simulink model "arm_model_pid"  (Simulink 7.7)
settings: Solver=ode4  StartTime=0.0  StopTime=1  FixedStep=1e-3  RelTol=1e-3
values from neighbouring files (symbols this model uses):
  dest = find_ik_solution(target,[L1,L2])    [init_param.m]
  g = 9.81    [init_param.m]    (also in nms_model_MechInit.m)
  L1 = 0.28    [init_param.m]
  L2 = 0.32    [init_param.m]
  N = 1.5    [muscleParams.m]    (also in nms_model_MechInit.m)
  s = orProblemSendCommand(['LoadIKFastSolver robot Translation3D'],probid)    [init.m]
libraries: mblibv1 x17, simulink x5
settings Model: Creator=icoderaven  LastModifiedBy=icoderaven
settings DataIOCC: SignalLoggingSaveFormat=Dataset
settings OptimizationCC: ExpressionDepthLimit=128
settings DebuggingCC: FcnCallInpInsideContextMsg=Enable All
settings CodeAppCC: CustomSymbolStrType=$N$R$M_T
settings GRTTargetCC: CombineOutputUpdateFcns=on
settings SimMechanicsCC: VisOnUpdateDiagram=on  VisDuringSimulation=on
settings ConfigurationSet: Description=SimMechanics 2G

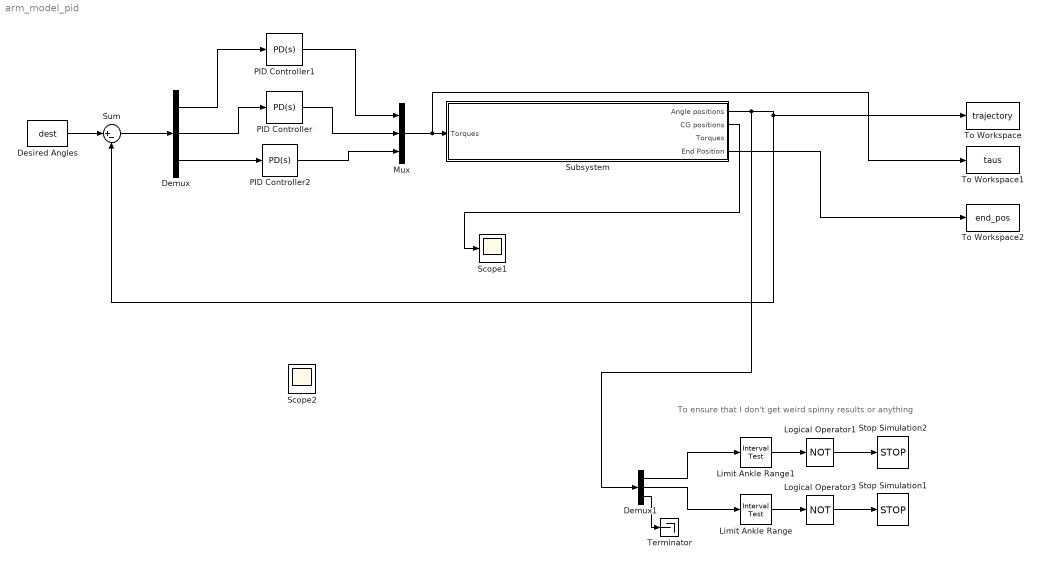
== system arm_model_pid ==
  note: To ensure that I don't get weird spinny results or anything
  Demux : Demux  Outputs=3
  Demux1 : Demux  Outputs=3
  Desired Angles : Constant  Value=dest
  Limit Ankle Range : simulink/Logic and Bit Operations/Interval Test  IntervalClosedRight=on  uplimit=150*pi/180  IntervalClosedLeft=on  lowlimit=0*pi/180  LogicOutDataTypeMode=boolean
  Limit Ankle Range1 : simulink/Logic and Bit Operations/Interval Test  IntervalClosedRight=on  uplimit=180*pi/180  IntervalClosedLeft=on  lowlimit=-45*pi/180  LogicOutDataTypeMode=boolean
  Logical Operator1 : Logic  Operator=NOT  AllPortsSameDT=off  OutDataTypeStr=boolean
  Logical Operator3 : Logic  Operator=NOT  AllPortsSameDT=off  OutDataTypeStr=boolean
  Mux : Mux  Inputs=3
  PID Controller : simulink/Continuous/PID Controller  Controller=PD  TimeDomain=Continuous-time  SampleTime=1  IntegratorMethod=Forward Euler  FilterMethod=Forward Euler  Form=Parallel  P=34.6616213286309  I=0.219466074591108  D=6.99160554908179  N=51.5441934181628  InitialConditionSource=internal  InitialConditionForIntegrator=0  InitialConditionForFilter=0  ExternalReset=none  LimitOutput=on  UpperSaturationLimit=200  LowerSaturationLimit=-200  LinearizeAsGain=off  AntiWindupMode=none  Kb=1  TrackingMode=off  Kt=1  PParamMin=[]  PParamMax=[]  IParamMin=[]  IParamMax=[]  DParamMin=[]  DParamMax=[]  NParamMin=[]  NParamMax=[]  KbParamMin=[]  KbParamMax=[]  KtParamMin=[]  KtParamMax=[]  POutMin=[]  POutMax=[]  IOutMin=[]  IOutMax=[]  DOutMin=[]  DOutMax=[]  NOutMin=[]  NOutMax=[]  KbOutMin=[]  KbOutMax=[]  KtOutMin=[]  KtOutMax=[]  IntegratorOutMin=[]  IntegratorOutMax=[]  FilterOutMin=[]  FilterOutMax=[]  SumOutMin=[]  SumOutMax=[]  SumI1OutMin=[]  SumI1OutMax=[]  SumI2OutMin=[]  SumI2OutMax=[]  SumI3OutMin=[]  SumI3OutMax=[]  SumDOutMin=[]  SumDOutMax=[]  SaturationOutMin=[]  SaturationOutMax=[]  IntegratorContinuousStateAttributes=''  IntegratorStateMustResolveToSignalObject=off  IntegratorRTWStateStorageClass=Auto  FilterContinuousStateAttributes=''  FilterStateMustResolveToSignalObject=off  FilterRTWStateStorageClass=Auto
  PID Controller1 : simulink/Continuous/PID Controller  Controller=PD  TimeDomain=Continuous-time  SampleTime=1  IntegratorMethod=Forward Euler  FilterMethod=Forward Euler  Form=Parallel  P=74.4712745992682  I=15180.7317223686  D=10.4723028081317  N=27.129113033617  InitialConditionSource=internal  InitialConditionForIntegrator=0  InitialConditionForFilter=0  ExternalReset=none  LimitOutput=on  UpperSaturationLimit=200  LowerSaturationLimit=-200  LinearizeAsGain=off  AntiWindupMode=none  Kb=1  TrackingMode=off  Kt=1  PParamMin=[]  PParamMax=[]  IParamMin=[]  IParamMax=[]  DParamMin=[]  DParamMax=[]  NParamMin=[]  NParamMax=[]  KbParamMin=[]  KbParamMax=[]  KtParamMin=[]  KtParamMax=[]  POutMin=[]  POutMax=[]  IOutMin=[]  IOutMax=[]  DOutMin=[]  DOutMax=[]  NOutMin=[]  NOutMax=[]  KbOutMin=[]  KbOutMax=[]  KtOutMin=[]  KtOutMax=[]  IntegratorOutMin=[]  IntegratorOutMax=[]  FilterOutMin=[]  FilterOutMax=[]  SumOutMin=[]  SumOutMax=[]  SumI1OutMin=[]  SumI1OutMax=[]  SumI2OutMin=[]  SumI2OutMax=[]  SumI3OutMin=[]  SumI3OutMax=[]  SumDOutMin=[]  SumDOutMax=[]  SaturationOutMin=[]  SaturationOutMax=[]  IntegratorContinuousStateAttributes=''  IntegratorStateMustResolveToSignalObject=off  IntegratorRTWStateStorageClass=Auto  FilterContinuousStateAttributes=''  FilterStateMustResolveToSignalObject=off  FilterRTWStateStorageClass=Auto
  PID Controller2 : simulink/Continuous/PID Controller  Controller=PD  TimeDomain=Continuous-time  SampleTime=1  IntegratorMethod=Forward Euler  FilterMethod=Forward Euler  Form=Parallel  P=5.74233404990851  I=38.1400991342515  D=65.6199753295884  N=1142.8279760416  InitialConditionSource=internal  InitialConditionForIntegrator=0  InitialConditionForFilter=0  ExternalReset=none  LimitOutput=on  UpperSaturationLimit=200  LowerSaturationLimit=-200  LinearizeAsGain=on  AntiWindupMode=none  Kb=1  TrackingMode=off  Kt=1  PParamMin=[]  PParamMax=[]  IParamMin=[]  IParamMax=[]  DParamMin=[]  DParamMax=[]  NParamMin=[]  NParamMax=[]  KbParamMin=[]  KbParamMax=[]  KtParamMin=[]  KtParamMax=[]  POutMin=[]  POutMax=[]  IOutMin=[]  IOutMax=[]  DOutMin=[]  DOutMax=[]  NOutMin=[]  NOutMax=[]  KbOutMin=[]  KbOutMax=[]  KtOutMin=[]  KtOutMax=[]  IntegratorOutMin=[]  IntegratorOutMax=[]  FilterOutMin=[]  FilterOutMax=[]  SumOutMin=[]  SumOutMax=[]  SumI1OutMin=[]  SumI1OutMax=[]  SumI2OutMin=[]  SumI2OutMax=[]  SumI3OutMin=[]  SumI3OutMax=[]  SumDOutMin=[]  SumDOutMax=[]  SaturationOutMin=[]  SaturationOutMax=[]  IntegratorContinuousStateAttributes=''  IntegratorStateMustResolveToSignalObject=off  IntegratorRTWStateStorageClass=Auto  FilterContinuousStateAttributes=''  FilterStateMustResolveToSignalObject=off  FilterRTWStateStorageClass=Auto
  Scope1 : Scope
      settings: YMin=-1.3  YMax=0  SaveName=ScopeData4
  Scope2 : Scope  NumInputPorts=6
      settings: YMin=-1.3~-5~-5~-5~-5~-5  YMax=0~5~5~5~5~5  SaveName=ScopeData5
  Stop Simulation1 : Stop
  Stop Simulation2 : Stop
  Subsystem : Subsystem
  Sum : Sum  Inputs=|+-
  Terminator : Terminator
  To Workspace : ToWorkspace  VariableName=trajectory  SampleTime=-1  SaveFormat=Structure With Time
  To Workspace1 : ToWorkspace  VariableName=taus  SampleTime=-1  SaveFormat=Structure With Time
  To Workspace2 : ToWorkspace  VariableName=end_pos  SampleTime=-1  SaveFormat=Structure With Time
  wires:
  Mux/1 -> To Workspace1/1, Subsystem/1("Torques ")
  Sum/1 -> Demux/1
  PID Controller/1 -> Mux/2
  Demux/3 -> PID Controller2/1
  Demux/2 -> PID Controller/1
  Demux/1 -> PID Controller1/1
  PID Controller1/1 -> Mux/1
  PID Controller2/1 -> Mux/3
  Subsystem/2("CG positions ") -> Scope1/1
  Desired Angles/1 -> Sum/1
  Subsystem/4(End Position) -> To Workspace2/1
  Subsystem/1(Angle positions) -> Demux1/1, Sum/2, To Workspace/1
  Limit Ankle Range/1 -> Logical Operator3/1
  Logical Operator3/1 -> Stop Simulation1/1
  Limit Ankle Range1/1 -> Logical Operator1/1
  Logical Operator1/1 -> Stop Simulation2/1
  Demux1/1 -> Limit Ankle Range1/1
  Demux1/2 -> Limit Ankle Range/1
  Demux1/3 -> Terminator/1

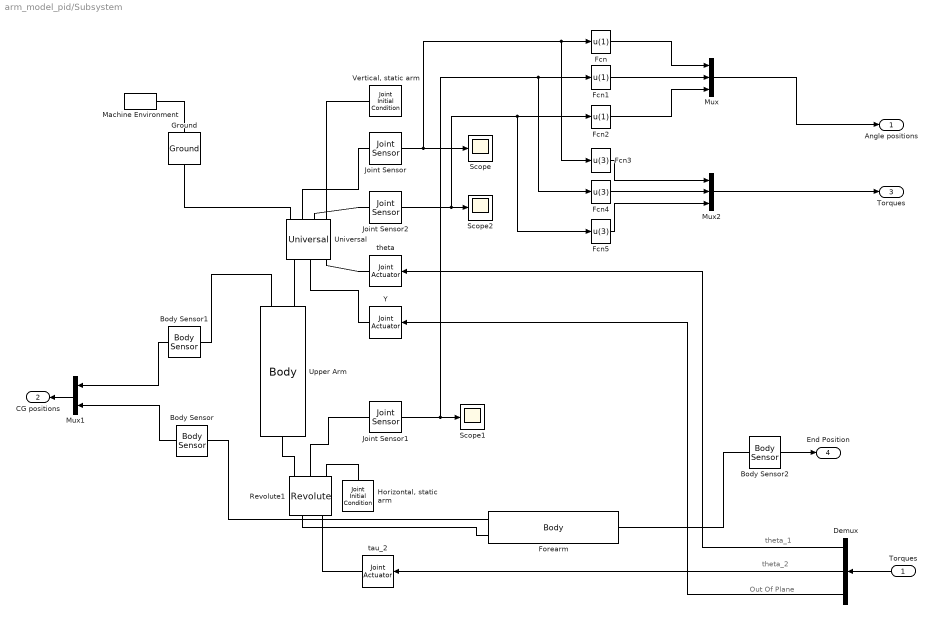
== system arm_model_pid/Subsystem ==
  note: theta_2
  note: theta_1
  note: Out Of Plane
  "Torques " : Inport
  Body Sensor : mblibv1/Sensors &  Actuators/Body Sensor  UpdateFromCAD=off  PhysicalDomain=Mechanical  PortType=blob  Muxed=on  Pose=off  Angle=on  AngleUnits=deg  ArcVelocity=off  ArcVelocityUnits=deg/s  ArcAcceleration=off  ArcAccelerationUnits=deg/s^2  CoordPosition=on  CoordPositionUnits=m  Velocity=off  VelocityUnits=m/s  Acceleration=off  AccelerationUnits=m/s^2  Quaternion=on  QuaternionDT=off  QuaternionDDT=off  QuaternionUnits=off  OutputVector=[1]  ActiveIO=on  Width=3  DialogClass=MechanicalSensorBlock  ReferenceFrame=Absolute (World)
  Body Sensor1 : mblibv1/Sensors &  Actuators/Body Sensor  UpdateFromCAD=off  PhysicalDomain=Mechanical  PortType=blob  Muxed=on  Pose=off  Angle=on  AngleUnits=deg  ArcVelocity=off  ArcVelocityUnits=deg/s  ArcAcceleration=off  ArcAccelerationUnits=deg/s^2  CoordPosition=on  CoordPositionUnits=m  Velocity=off  VelocityUnits=m/s  Acceleration=off  AccelerationUnits=m/s^2  Quaternion=on  QuaternionDT=off  QuaternionDDT=off  QuaternionUnits=off  OutputVector=[1]  ActiveIO=on  Width=3  DialogClass=MechanicalSensorBlock  ReferenceFrame=Absolute (World)
  Body Sensor2 : mblibv1/Sensors &  Actuators/Body Sensor  UpdateFromCAD=off  PhysicalDomain=Mechanical  PortType=blob  Muxed=on  Pose=off  Angle=on  AngleUnits=deg  ArcVelocity=off  ArcVelocityUnits=deg/s  ArcAcceleration=off  ArcAccelerationUnits=deg/s^2  CoordPosition=on  CoordPositionUnits=m  Velocity=off  VelocityUnits=m/s  Acceleration=off  AccelerationUnits=m/s^2  Quaternion=on  QuaternionDT=off  QuaternionDDT=off  QuaternionUnits=off  OutputVector=[1]  ActiveIO=on  Width=3  DialogClass=MechanicalSensorBlock  ReferenceFrame=Absolute (World)
  Demux : Demux  Outputs=3
  Fcn : Fcn  Expr=u(1)
  Fcn1 : Fcn  Expr=u(1)
  Fcn2 : Fcn  Expr=u(1)
  Fcn3 : Fcn  Expr=u(3)
  Fcn4 : Fcn  Expr=u(3)
  Fcn5 : Fcn  Expr=u(3)
  Forearm : mblibv1/Bodies/Body  LConnTagsString=CG|CS1  RConnTagsString=CS2  UpdateFromCAD=off  DialogClass=MechanicalBodyBlock  Mass=1  MassUnits=kg  InertiaUnits=kg*m^2  Inertia=eye(3)  Shape=Cylinder  ShapeDims=[1 1]  ShapeUnits=m  ShapeUse=false  Density=1  DensityUnits=kg/m^3  DensityUse=false  GraphicsMode=MACHINE_DEFAULT  BodyColorSelMode=MACHINE_DEFAULT  BodyColor=[1 0 0]  AttachedToCS=CG  CG=Left$CG$[0 -L2/2 0]$CS1$CS1$m$[0 0 0]$Euler X-Y-Z$deg$WORLD$true$none  WorkingFrames=Left$CS1$[0 0 0]$Adjoining$Adjoining$m$[0 0 0]$Euler X-Y-Z$deg$WORLD$true$none#Right$CS2$[0 -L2 0]$CS1$CS1$m$[0 0 0]$Euler X-Y-Z$deg$WORLD$true$none  CGPos=[0 -L2/2 0]  CGRot=[0 0 0]  CS0Pos=[]  CS0Rot=[]  CS1Pos=[0 0 0]  CS1Rot=[0 0 0]  CS2Pos=[0 -L2 0]  CS2Rot=[0 0 0]  CS3Pos=[]  CS3Rot=[]  CS4Pos=[]  CS4Rot=[]  CS5Pos=[]  CS5Rot=[]  CS6Pos=[]  CS6Rot=[]  CS7Pos=[]  CS7Rot=[]  CS8Pos=[]  CS8Rot=[]  CS9Pos=[]  CS9Rot=[]  CS10Pos=[]  CS10Rot=[]  CS11Pos=[]  CS11Rot=[]  CS12Pos=[]  CS12Rot=[]  CS13Pos=[]  CS13Rot=[]  CS14Pos=[]  CS14Rot=[]  CS15Pos=[]  CS15Rot=[]  CS16Pos=[]  CS16Rot=[]  CS17Pos=[]  CS17Rot=[]  CS18Pos=[]  CS18Rot=[]  CS19Pos=[]  CS19Rot=[]  CS20Pos=[]  CS20Rot=[]
  Ground : mblibv1/Bodies/Ground  UpdateFromCAD=off  LeftPortType=env  RightPortType=workingframe  PhysicalDomain=Mechanical  DialogClass=GroundBlock  CoordPosition=[0 0 0]  CoordPositionUnits=m  StateVectorMgrId=-1  MachineId=[0 0]  ShowEnvPort=on
  "Horizontal, static arm" : mblibv1/Sensors &  Actuators/Joint Initial Condition  UpdateFromCAD=off  LeftPortType=blob  RightPortType=blob  PhysicalDomain=mechanical  DialogClass=InitialConditionBlock  InitialConditions=P1$false$0$m$deg$0$m/s$deg/s#P2$false$0$m$deg$0$m/s$deg/s#P3$false$0$m$deg$0$m/s$deg/s#R1$false$0$m$deg$0$m/s$deg/s#R2$false$0$m$deg$0$m/s$deg/s#R3$false$0$m$deg$0$m/s$deg/s#S$false$0$m$deg$0$m/s$deg/s  P1PIC=0  P1VIC=0  P2PIC=0  P2VIC=0  P3PIC=0  P3VIC=0  R1PIC=0  R1VIC=0  R2PIC=0  R2VIC=0  R3PIC=0  R3VIC=0  SPIC=0  SVIC=0
  Joint Sensor : mblibv1/Sensors &  Actuators/Joint Sensor  UpdateFromCAD=off  PhysicalDomain=Mechanical  PortType=blob  Muxed=on  Pose=off  Angle=on  AngleUnits=rad  ArcVelocity=on  ArcVelocityUnits=rad/s  ArcAcceleration=off  ArcAccelerationUnits=deg/s^2  CoordPosition=on  CoordPositionUnits=m  Velocity=off  VelocityUnits=m/s  Acceleration=off  AccelerationUnits=m/s^2  Quaternion=on  QuaternionDT=off  QuaternionDDT=off  QuaternionUnits=off  OutputVector=[1]  ActiveIO=on  Width=3  DialogClass=MechanicalSensorBlock  Primitive=R1  Force=off  ForceUnits=N  Torque=on  TorqueUnits=N*m  ReferenceFrame=Absolute (World)  ReactionSensedSide=Base  ReactionReferenceFrame=Absolute (World)  ReactionForce=off  ReactionForceUnits=N  ReactionMoment=off  ReactionMomentUnits=N*m
  Joint Sensor1 : mblibv1/Sensors &  Actuators/Joint Sensor  UpdateFromCAD=off  PhysicalDomain=Mechanical  PortType=blob  Muxed=on  Pose=off  Angle=on  AngleUnits=rad  ArcVelocity=on  ArcVelocityUnits=rad/s  ArcAcceleration=off  ArcAccelerationUnits=deg/s^2  CoordPosition=on  CoordPositionUnits=m  Velocity=off  VelocityUnits=m/s  Acceleration=off  AccelerationUnits=m/s^2  Quaternion=on  QuaternionDT=off  QuaternionDDT=off  QuaternionUnits=off  OutputVector=[1]  ActiveIO=on  Width=3  DialogClass=MechanicalSensorBlock  Primitive=R1  Force=off  ForceUnits=N  Torque=on  TorqueUnits=N*m  ReferenceFrame=Absolute (World)  ReactionSensedSide=Base  ReactionReferenceFrame=Absolute (World)  ReactionForce=off  ReactionForceUnits=N  ReactionMoment=off  ReactionMomentUnits=N*m
  Joint Sensor2 : mblibv1/Sensors &  Actuators/Joint Sensor  UpdateFromCAD=off  PhysicalDomain=Mechanical  PortType=blob  Muxed=on  Pose=off  Angle=on  AngleUnits=rad  ArcVelocity=on  ArcVelocityUnits=rad/s  ArcAcceleration=off  ArcAccelerationUnits=deg/s^2  CoordPosition=on  CoordPositionUnits=m  Velocity=off  VelocityUnits=m/s  Acceleration=off  AccelerationUnits=m/s^2  Quaternion=on  QuaternionDT=off  QuaternionDDT=off  QuaternionUnits=off  OutputVector=[1]  ActiveIO=on  Width=3  DialogClass=MechanicalSensorBlock  Primitive=R2  Force=off  ForceUnits=N  Torque=on  TorqueUnits=N*m  ReferenceFrame=Absolute (World)  ReactionSensedSide=Base  ReactionReferenceFrame=Absolute (World)  ReactionForce=off  ReactionForceUnits=N  ReactionMoment=off  ReactionMomentUnits=N*m
  Machine Environment : mblibv1/Bodies/Machine Environment  PortType=env  PhysicalDomain=Mechanical  DialogTemplateClass=MECH.MachineEnvironment  SyncWhenCopied=off  Gravity=[0 -g 0]  GravityUnits=m/s^2  GravityAsSignal=off  Dimensionality=Auto-detect  AnalysisType=Forward dynamics  LinearAssemblyTolerance=1e-3  LinearAssemblyToleranceUnits=m  AngularAssemblyTolerance=1e-3  AngularAssemblyToleranceUnits=rad  ConstraintSolverType=Stabilizing  ConstraintRelTolerance=1e-4  ConstraintAbsTolerance=1e-4  UseRobustSingularityHandling=off  RedundancyAnalysisToleranceType=Automatically select tolerance  RedundancyAnalysisTolerance=1e-14  StatePerturbationType=Fixed  PerturbationSize=1e-5  VisualizeMachine=on  BodyVisualizationType=Use model default body geometries  BodyColorSelMode=Use model default  DefaultBodyColor=[1 0 0]
  Mux : Mux  Inputs=3
  Mux1 : Mux  Inputs=2
  Mux2 : Mux  Inputs=3
  Revolute1 : mblibv1/Joints/Revolute  LConnTagsString=__newl0|SA1|SA2  RConnTagsString=__newr0|SA1  UpdateFromCAD=off  NumSAPorts=3  CutJoint=off  MarkAsCut=off  Primitives=prismatic  PrimitiveProps=R1$World$[0 0 1]$revolute  DialogClass=JointBlock  R1Axis=[0 0 1]
  Scope : Scope
  Scope1 : Scope
  Scope2 : Scope
      settings: SaveName=ScopeData2
  Universal : mblibv1/Joints/Universal  LConnTagsString=__newl0|SA1|SA2|SA3  RConnTagsString=__newr0|SA1|SA2  UpdateFromCAD=off  NumSAPorts=5  CutJoint=off  MarkAsCut=off  Primitives=prismatic  PrimitiveProps=R1$World$[0 0 1]$revolute#R2$World$[1 0 0]$revolute  DialogClass=JointBlock  R1Axis=[0 0 1]  R2Axis=[1 0 0]
  Upper Arm : mblibv1/Bodies/Body  LConnTagsString=CG|CS1  RConnTagsString=CS2  UpdateFromCAD=off  DialogClass=MechanicalBodyBlock  Mass=1  MassUnits=kg  InertiaUnits=kg*m^2  Inertia=eye(3)  Shape=Cylinder  ShapeDims=[1 1]  ShapeUnits=m  ShapeUse=false  Density=1  DensityUnits=kg/m^3  DensityUse=false  GraphicsMode=MACHINE_DEFAULT  BodyColorSelMode=MACHINE_DEFAULT  BodyColor=[1 0 0]  AttachedToCS=CG  CG=Left$CG$[0 -L1/2 0]$CS1$CS1$m$[0 0 0]$Euler X-Y-Z$deg$WORLD$true$none  WorkingFrames=Left$CS1$[0 0 0]$World$World$m$[0 0 0]$Euler X-Y-Z$deg$WORLD$true$none#Right$CS2$[0 -L1 0]$CS1$CS1$m$[0 0 0]$Euler X-Y-Z$deg$WORLD$true$none  CGPos=[0 -L1/2 0]  CGRot=[0 0 0]  CS0Pos=[]  CS0Rot=[]  CS1Pos=[0 0 0]  CS1Rot=[0 0 0]  CS2Pos=[0 -L1 0]  CS2Rot=[0 0 0]  CS3Pos=[]  CS3Rot=[]  CS4Pos=[]  CS4Rot=[]  CS5Pos=[]  CS5Rot=[]  CS6Pos=[]  CS6Rot=[]  CS7Pos=[]  CS7Rot=[]  CS8Pos=[]  CS8Rot=[]  CS9Pos=[]  CS9Rot=[]  CS10Pos=[]  CS10Rot=[]  CS11Pos=[]  CS11Rot=[]  CS12Pos=[]  CS12Rot=[]  CS13Pos=[]  CS13Rot=[]  CS14Pos=[]  CS14Rot=[]  CS15Pos=[]  CS15Rot=[]  CS16Pos=[]  CS16Rot=[]  CS17Pos=[]  CS17Rot=[]  CS18Pos=[]  CS18Rot=[]  CS19Pos=[]  CS19Rot=[]  CS20Pos=[]  CS20Rot=[]
  "Vertical, static arm" : mblibv1/Sensors &  Actuators/Joint Initial Condition  UpdateFromCAD=off  LeftPortType=blob  RightPortType=blob  PhysicalDomain=mechanical  DialogClass=InitialConditionBlock  InitialConditions=P1$false$0$m$deg$0$m/s$deg/s#P2$false$0$m$deg$0$m/s$deg/s#P3$false$0$m$deg$0$m/s$deg/s#R1$true$0$m$deg$0$m/s$deg/s#R2$true$0$m$deg$0$m/s$deg/s#R3$false$0$m$deg$0$m/s$deg/s#S$false$0$m$deg$0$m/s$deg/s  P1PIC=0  P1VIC=0  P2PIC=0  P2VIC=0  P3PIC=0  P3VIC=0  R1PIC=0  R1VIC=0  R2PIC=0  R2VIC=0  R3PIC=0  R3VIC=0  SPIC=0  SVIC=0
  Y : mblibv1/Sensors &  Actuators/Joint Actuator  UpdateFromCAD=off  PhysicalDomain=Mechanical  PortType=blob  ActuationStyle=Force  AngleUnits=deg  ArcVelocityUnits=deg/s  ArcAccelerationUnits=deg/s^2  CoordPositionUnits=m  VelocityUnits=m/s  AccelerationUnits=m/s^2  ForceUnits=N  TorqueUnits=N*m  ActiveIO=on  Width=1  DialogClass=MechanicalActuatorBlock  Primitive=R2  ReferenceFrame=Absolute (World)
  tau_2 : mblibv1/Sensors &  Actuators/Joint Actuator  UpdateFromCAD=off  PhysicalDomain=Mechanical  PortType=blob  ActuationStyle=Force  AngleUnits=deg  ArcVelocityUnits=deg/s  ArcAccelerationUnits=deg/s^2  CoordPositionUnits=m  VelocityUnits=m/s  AccelerationUnits=m/s^2  ForceUnits=N  TorqueUnits=N*m  ActiveIO=on  Width=1  DialogClass=MechanicalActuatorBlock  Primitive=R1  ReferenceFrame=Absolute (World)
  theta : mblibv1/Sensors &  Actuators/Joint Actuator  UpdateFromCAD=off  PhysicalDomain=Mechanical  PortType=blob  ActuationStyle=Force  AngleUnits=deg  ArcVelocityUnits=deg/s  ArcAccelerationUnits=deg/s^2  CoordPositionUnits=m  VelocityUnits=m/s  AccelerationUnits=m/s^2  ForceUnits=N  TorqueUnits=N*m  ActiveIO=on  Width=1  DialogClass=MechanicalActuatorBlock  Primitive=R1  ReferenceFrame=Absolute (World)
  Angle positions : Outport
  "CG positions " : Outport  Port=2
  Torques : Outport  Port=3
  End Position : Outport  Port=4
  wires:
  Demux/3 -> Y/1
  Demux/2 -> tau_2/1
  Joint Sensor/1 -> Fcn3/1, Fcn/1, Scope/1
  Joint Sensor1/1 -> Fcn4/1, Fcn1/1, Scope1/1
  Demux/1 -> theta/1
  Joint Sensor2/1 -> Fcn5/1, Fcn2/1, Scope2/1
  "Torques "/1 -> Demux/1
  Mux/1 -> Angle positions/1
  Fcn/1 -> Mux/1
  Fcn1/1 -> Mux/2
  Fcn2/1 -> Mux/3
  Body Sensor/1 -> Mux1/2
  Mux1/1 -> "CG positions "/1
  Body Sensor1/1 -> Mux1/1
  Mux2/1 -> Torques/1
  Fcn3/1 -> Mux2/1
  Fcn4/1 -> Mux2/2
  Fcn5/1 -> Mux2/3
  Body Sensor2/1 -> End Position/1
  connections:
  Universal/LConn1 -- Ground/RConn1
  Universal/RConn1 -- Upper Arm/LConn2
  Revolute1/LConn1 -- Upper Arm/RConn1
  Revolute1/RConn1 -- Forearm/LConn2
  Machine Environment/RConn1 -- Ground/LConn1
  Universal/LConn2 -- Joint Sensor/LConn1
  Universal/RConn2 -- Y/RConn1
  tau_2/RConn1 -- Revolute1/RConn2
  Joint Sensor1/LConn1 -- Revolute1/LConn2
  theta/RConn1 -- Universal/RConn3
  Joint Sensor2/LConn1 -- Universal/LConn3
  "Vertical, static arm"/RConn1 -- Universal/LConn4
  Revolute1/LConn3 -- "Horizontal, static arm"/RConn1
  Body Sensor/LConn1 -- Forearm/LConn1
  Upper Arm/LConn1 -- Body Sensor1/LConn1
  Body Sensor2/LConn1 -- Forearm/RConn1
